simulink model "matlab2018b"  (R2024a)
settings: Solver=ode4  StartTime=0.0  StopTime=10.0  FixedStep=0.005  RelTol=1e-3
settings Model: Creator=RIver  LastModifiedBy=郑家浩
settings SolverCC: AlgebraicLoopSolver=TrustRegion
settings DataIOCC: ReturnWorkspaceOutputs=off
settings DebuggingCC: UnconnectedInputMsg=warning  UnconnectedOutputMsg=warning  UnconnectedLineMsg=warning  ArithmeticOperatorsInVariantConditions=warning
settings ModelReferenceCC: EnableRefExpFcnMdlSchedulingChecks=on
settings SFSimCC: CustomCodeUndefinedFunction=UseInterfaceOnly
settings RTWCC: GPUComputeCapability=3.5

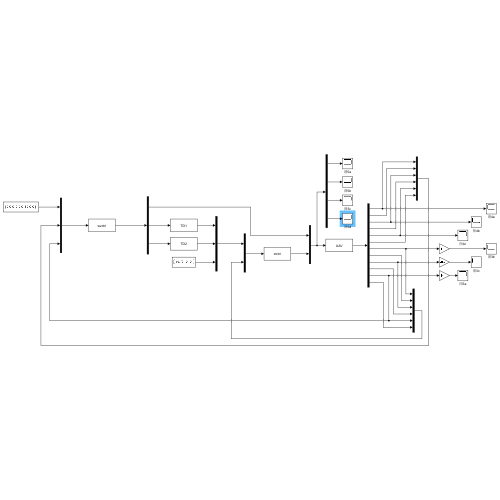
[thumbnail: Simulink's stored preview of the top-level diagram]
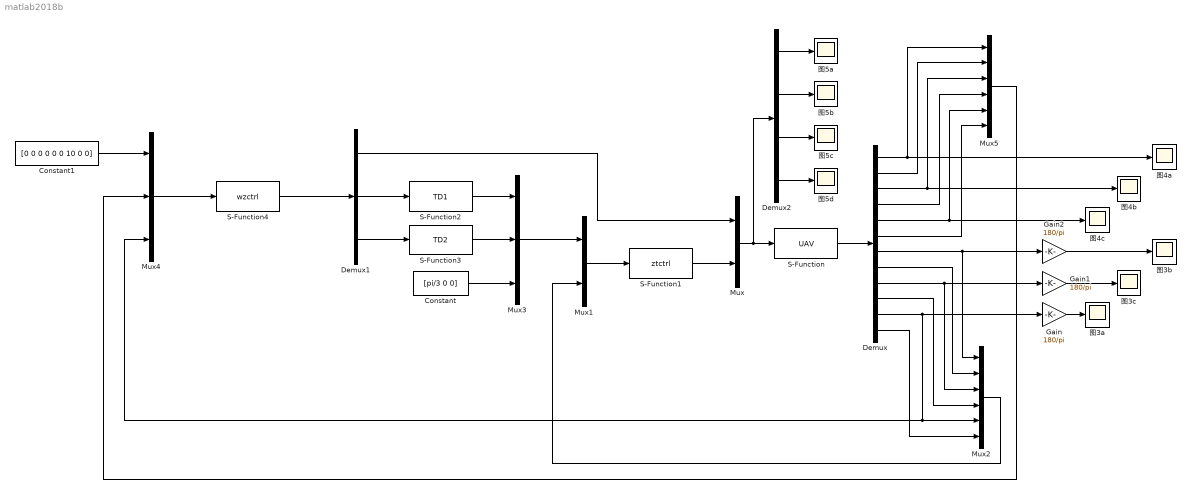
== system matlab2018b ==
  Constant : Constant  Value=[pi/3 0 0]
  Constant1 : Constant  Value=[0 0 0 0 0 0 10 0 0]
  Demux : Demux  Outputs=12
  Demux1 : Demux  Outputs=3
  Demux2 : Demux
  Gain : Gain  Gain=180/pi
  Gain1 : Gain  Gain=180/pi
  Gain2 : Gain  Gain=180/pi
  Mux : Mux  Inputs=2
  Mux1 : Mux  Inputs=2
  Mux2 : Mux  Inputs=6
  Mux3 : Mux  Inputs=3
  Mux4 : Mux  Inputs=3
  Mux5 : Mux  Inputs=6
  S-Function : S-Function  FunctionName=UAV  SFunctionDeploymentMode=off  EnableBusSupport=off
  S-Function1 : S-Function  FunctionName=ztctrl  SFunctionDeploymentMode=off  EnableBusSupport=off
  S-Function2 : S-Function  FunctionName=TD1  SFunctionDeploymentMode=off  EnableBusSupport=off
  S-Function3 : S-Function  FunctionName=TD2  SFunctionDeploymentMode=off  EnableBusSupport=off
  S-Function4 : S-Function  FunctionName=wzctrl  SFunctionDeploymentMode=off  EnableBusSupport=off
  图3a : Scope
  图3b : Scope
  图3c : Scope
  图4a : Scope
  图4b : Scope
  图4c : Scope
  图5a : Scope
  图5b : Scope
  图5c : Scope
  图5d : Scope
  wires:
  Mux/1 -> Demux2/1, S-Function/1
  S-Function/1 -> Demux/1
  Demux/1 -> 图4a/1, Mux5/1
  Demux/3 -> Mux5/3, 图4b/1
  Demux/5 -> Mux5/5, 图4c/1
  Demux/7 -> Mux2/1, Gain2/1
  Demux/9 -> Mux2/3, Gain1/1
  S-Function1/1 -> Mux/2
  Mux1/1 -> S-Function1/1
  Demux/8 -> Mux2/2
  Demux/10 -> Mux2/4
  Demux/12 -> Mux2/6
  Mux2/1 -> Mux1/2
  Mux3/1 -> Mux1/1
  Constant/1 -> Mux3/3
  S-Function2/1 -> Mux3/1
  S-Function3/1 -> Mux3/2
  Demux1/1 -> Mux/1
  Demux1/2 -> S-Function2/1
  Demux1/3 -> S-Function3/1
  Mux5/1 -> Mux4/2
  Constant1/1 -> Mux4/1
  Demux/11 -> Mux4/3, Mux2/5, Gain/1
  S-Function4/1 -> Demux1/1
  Mux4/1 -> S-Function4/1
  Demux/2 -> Mux5/2
  Demux/4 -> Mux5/4
  Demux/6 -> Mux5/6
  Demux2/1 -> 图5a/1
  Demux2/2 -> 图5b/1
  Demux2/3 -> 图5c/1
  Demux2/4 -> 图5d/1
  Gain/1 -> 图3a/1
  Gain1/1 -> 图3c/1
  Gain2/1 -> 图3b/1
